simulink model "control_loop"  (R2023b)
settings: Solver=ode45  StartTime=0.0  StopTime=250  RelTol=1e-3
values from neighbouring files (symbols this model uses):
  alfa1 = 40    [vehicle_params.m]
  alfa2 = 35    [vehicle_params.m]
  alfa3 = 16    [vehicle_params.m]
  alfa4 = 12    [vehicle_params.m]
  alfa5 = 10    [vehicle_params.m]
  m = 1200    [vehicle_params.m]
libraries: slpidlib x1
(part 3 of 3)

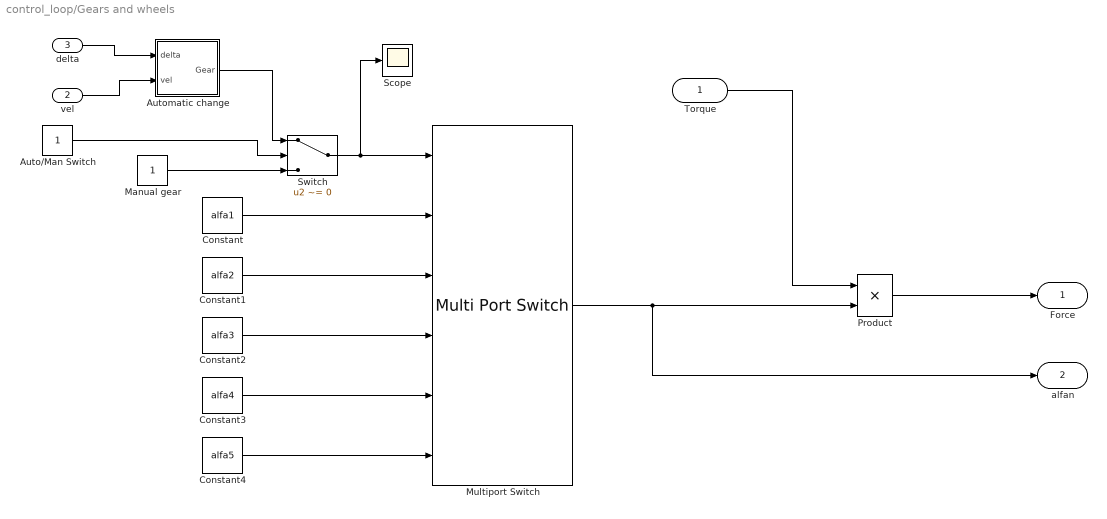
== system control_loop/Gears and wheels ==
  Torque : Inport
  vel : Inport  Port=2
  delta : Inport  Port=3
  Auto/Man Switch : Constant
  Automatic change : Stateflow chart  TreatAsAtomicUnit=on
  Constant : Constant  Value=alfa1
  Constant1 : Constant  Value=alfa2
  Constant2 : Constant  Value=alfa3
  Constant3 : Constant  Value=alfa4
  Constant4 : Constant  Value=alfa5
  Manual gear : Constant
  Multiport Switch : MultiPortSwitch  Inputs=5  SaturateOnIntegerOverflow=off  InputSameDT=off
  Product : Product
  Scope : Scope
  Switch : Switch  Criteria=u2 ~= 0  SaturateOnIntegerOverflow=off  InputSameDT=off
  Force : Outport
  alfan : Outport  Port=2
  wires:
  Multiport Switch/1 -> alfan/1, Product/2
  Constant/1 -> Multiport Switch/2
  Constant1/1 -> Multiport Switch/3
  Constant2/1 -> Multiport Switch/4
  Constant3/1 -> Multiport Switch/5
  Constant4/1 -> Multiport Switch/6
  Torque/1 -> Product/1
  Product/1 -> Force/1
  vel/1 -> Automatic change/2(vel)
  Automatic change/1(Gear) -> Switch/1
  Manual gear/1 -> Switch/3
  Auto/Man Switch/1 -> Switch/2
  delta/1 -> Automatic change/1(delta)
  Switch/1 -> Multiport Switch/1, Scope/1

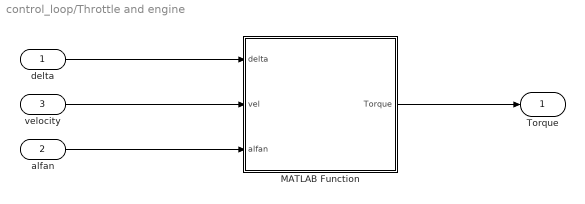
== system control_loop/Throttle and engine ==
  delta : Inport
  alfan : Inport  Port=2
  velocity : Inport  Port=3
  MATLAB Function : MATLAB Function  TreatAsAtomicUnit=on
  Torque : Outport
  wires:
  MATLAB Function/1(Torque) -> Torque/1
  delta/1 -> MATLAB Function/1(delta)
  velocity/1 -> MATLAB Function/2(vel)
  alfan/1 -> MATLAB Function/3(alfan)

== matlab function control_loop/Disturbance Force/MATLAB Function ==
  data: vel input; Fd output; theta input
function Fd = fcn(vel,theta)

% Parametrs

m       =   1200;    % Kg
g       =   9.81;    % m/s^2
Cr      =   0.01;
rho     =   1.3;     % kg/m^2
Cd      =   0.36;
A       =   2.2;     % m^2 

% Forces


Fd1 =   m*g*sin(theta);

Fd2 =   m*g*Cr*cos(theta)*sign(vel);

Fd3 =   1/2*rho*Cd*A*vel^2;



Fd = Fd1+Fd2+Fd3;

== stateflow chart control_loop/Gears and wheels/Automatic change ==
  state Second
    Gear=2;
  state Third
    Gear=3;
  state First
    Gear=1;
  state Fifth
    Gear=5;
  state Fourth
    Gear=4;
  Second -> Third [order 1] : [vel>=t2(delta)]
  First -> Second : [vel>=t1(delta)]
  Third -> Second [order 2] : [vel<t2(delta)]
  Second -> First [order 2] : [vel<t1(delta)]
  Third -> Fourth [order 1] : [vel>=t3(delta)]
  Fourth -> Third [order 2] : [vel<t3(delta)]
  (default) -> First
  Fifth -> Fourth : [vel<t4(delta)]
  Fourth -> Fifth [order 1] : [vel>=t4(delta)]
  data: a function_output; delta function_input; delta function_input; b function_output; delta function_input; c function_output; delta function_input; d function_output; delta input; Gear output; vel input; UP4 local; UP3 local; UP2 local; UP1 local; DOWN5 local; DOWN4 local; DOWN3 local; DOWN2 local
  function a=t1(delta):
    | function a=t1(delta)
    | 
    | % UP1/DOWN2
    | 
    | a=10.1042*delta^3+8.1875*delta^2-2.3917*delta+4.5;
    | 
    | 
    | end
  function b=t2(delta):
    | function b=t2(delta)
    | % UP2/DOWN3
    | 
    | b=52.3958*delta^3-36.9375*delta^2+8.1417*delta+5.3;
    | 
    | end
  function c=t3(delta):
    | function c=t3(delta)
    | % UP3/DOWN4
    | 
    | c=42.6042*delta^3+5.4375*delta^2-5.2417*delta+11.6;
    | 
    | end
  function d=t4(delta):
    | 
    | function d=t4(delta)
    | 
    | % UP4/DOWN5
    | 
    | d=30.4687*delta^3+38.8438*delta^2-15.4125*delta+15.5;
    | 
    | end

== matlab function control_loop/Throttle and engine/MATLAB Function ==
  data: delta input; Torque output; vel input; alfan input
function Torque = fcn(delta,vel,alfan)
% Parametrs

Tm      =   200;     % Nm
wm      =   450;     % rad/s
beta    =   0.35;


w=vel*alfan;


Torque = delta*Tm*(1-beta*(w/wm-1)^2);
